simulink model "simulink_frequenza"  (R2026a)
settings: Solver=ode23tb  StopTime=100  MaxStep=1e-3
settings Model: Creator=matte  LastModifiedBy=matte

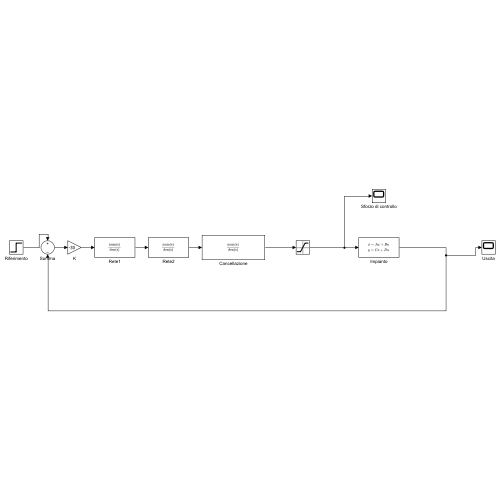
[thumbnail: Simulink's stored preview of the top-level diagram]
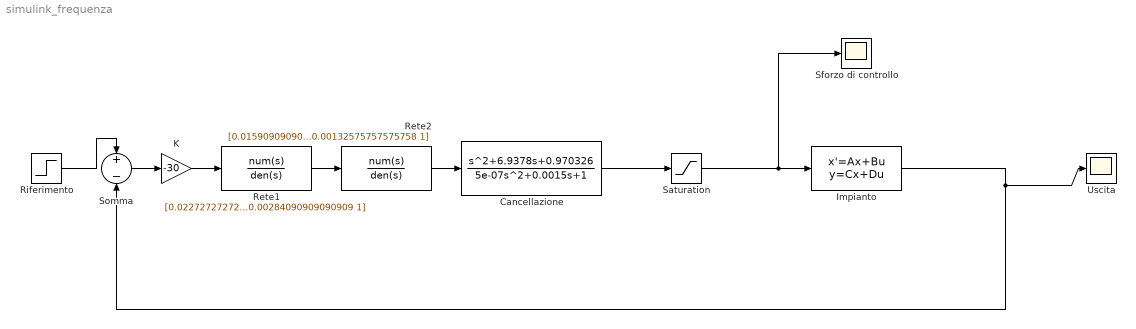
== system simulink_frequenza ==
  Cancellazione : TransferFcn  Numerator=[1 6.9378 0.970326]  Denominator=[5e-07 0.0015 1]
  Impianto : StateSpace  A=[0 1 0 0;0 -0.2 -3.924 0;0 0 0 1;0 0.666666666666667 45.78 0]  B=[0;2;0;-6.66666666666667]  C=[1 0 0.3 0]  D=0  InitialCondition=0
  K : Gain  Gain=-30
  Rete1 : TransferFcn  Numerator=[0.0227272727272727 1]  Denominator=[0.00284090909090909 1]
  Rete2 : TransferFcn  Numerator=[0.0159090909090909 1]  Denominator=[0.00132575757575758 1]
  Riferimento : Step  Time=0  SampleTime=0
  Saturation : Saturate  UpperLimit=10  LowerLimit=-10
  Sforzo di controllo : Scope
      settings: ActiveDisplayYMinimum=-3.9404184251564072  ActiveDisplayYMaximum=4.943098201470133
  Somma : Sum  Inputs=+-
  Uscita : Scope
      settings: ActiveDisplayYMinimum=-0.37189638669001668  ActiveDisplayYMaximum=1.1662098811434052
  wires:
  Riferimento/1 -> Somma/1
  Somma/1 -> K/1
  K/1 -> Rete1/1
  Rete1/1 -> Rete2/1
  Rete2/1 -> Cancellazione/1
  Impianto/1 -> Somma/2, Uscita/1
  Cancellazione/1 -> Saturation/1
  Saturation/1 -> Sforzo di controllo/1, Impianto/1
